simulink model "s0513_eARCmechfailflag_simplecomparison"  (R2021a)
settings: Solver=VariableStepAuto  StartTime=0.0  StopTime=10.0  RelTol=1e-3
libraries: CarMaker4SL x4
settings Model: Creator=jason  LastModifiedBy=jason

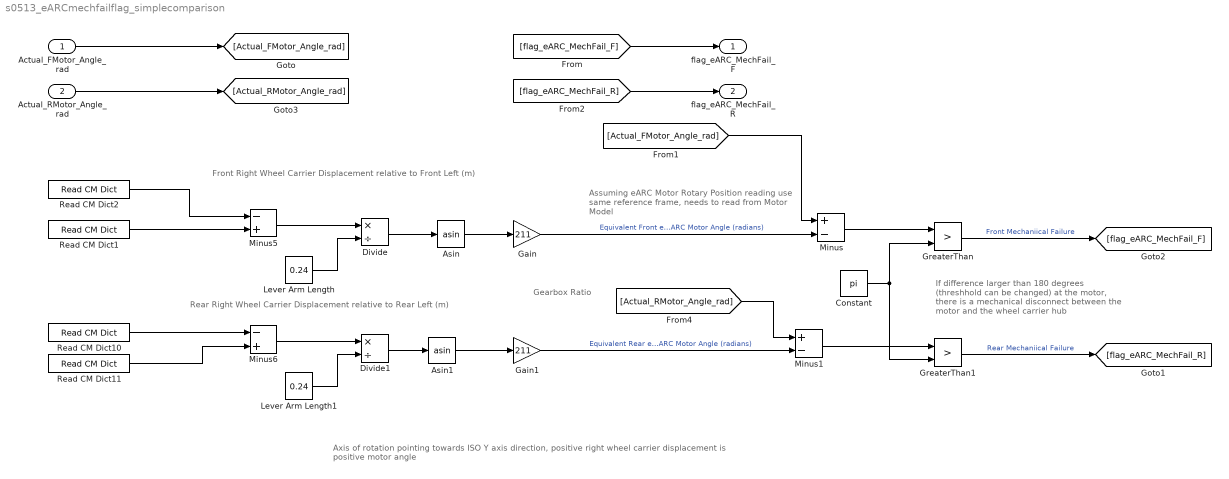
== system s0513_eARCmechfailflag_simplecomparison ==
  note: If difference larger than 180 degrees (threshhold can be changed) at the motor, there is a mechanical disconnect between the motor and the wheel carrier hub
  note: Assuming eARC Motor Rotary Position reading
      | use same reference frame, needs to read from Motor Model
  note: Axis of rotation pointing towards ISO Y axis direction, positive right wheel carrier displacement is positive motor angle
  note: Gearbox Ratio
  note: Rear Right Wheel Carrier Displacement relative to Rear Left (m)
  note: Front Right Wheel Carrier Displacement relative to Front Left (m)
  Actual_FMotor_Angle_rad : Inport
  Actual_RMotor_Angle_rad : Inport  Port=2
  Asin : Trigonometry  Operator=asin
  Asin1 : Trigonometry  Operator=asin
  Constant : Constant  Value=pi
  Divide : Product  Inputs=*/
  Divide1 : Product  Inputs=*/
  Gain : Gain  Gain=211
  Gain1 : Gain  Gain=211
  GreaterThan : RelationalOperator  Operator=>  OutDataTypeStr=boolean  RndMeth=Simplest
  GreaterThan1 : RelationalOperator  Operator=>  OutDataTypeStr=boolean  RndMeth=Simplest
  Lever Arm Length : Constant  Value=0.24
  Lever Arm Length1 : Constant  Value=0.24
  Minus : Sum  Inputs=+-
  Minus1 : Sum  Inputs=+-
  Minus5 : Sum  Inputs=-+
  Minus6 : Sum  Inputs=-+
  Read CM Dict1 : CarMaker4SL/Read CM Dict  xname=Car.CFR.q0  xsync=off  xstime=Continuous
  Read CM Dict10 : CarMaker4SL/Read CM Dict  xname=Car.CRL.q0  xsync=off  xstime=Continuous
  Read CM Dict11 : CarMaker4SL/Read CM Dict  xname=Car.CRR.q0  xsync=off  xstime=Continuous
  Read CM Dict2 : CarMaker4SL/Read CM Dict  xname=Car.CFL.q0  xsync=off  xstime=Continuous
  flag_eARC_MechFail_F : Outport
  flag_eARC_MechFail_R : Outport  Port=2
  wires:
  Minus6/1 -> Divide1/1
  Gain/1 -> Minus/2  "Equivalent Front eARC Motor Angle (radians)"
  Constant/1 -> GreaterThan1/2, GreaterThan/2
  Read CM Dict1/1 -> Minus5/2
  GreaterThan1/1 -> [flag_eARC_MechFail_R]  "Rear Mechaniical Failure"
  Gain1/1 -> Minus1/2  "Equivalent Rear eARC Motor Angle (radians)"
  GreaterThan/1 -> [flag_eARC_MechFail_F]  "Front Mechaniical Failure"
  Minus1/1 -> GreaterThan1/1
  [Actual_FMotor_Angle_rad] -> Minus/1
  [Actual_RMotor_Angle_rad] -> Minus1/1
  Lever Arm Length1/1 -> Divide1/2
  Lever Arm Length/1 -> Divide/2
  Divide1/1 -> Asin1/1
  Minus5/1 -> Divide/1
  Minus/1 -> GreaterThan/1
  Divide/1 -> Asin/1
  Read CM Dict2/1 -> Minus5/1
  Asin1/1 -> Gain1/1
  Asin/1 -> Gain/1
  Read CM Dict10/1 -> Minus6/1
  Read CM Dict11/1 -> Minus6/2
  Actual_FMotor_Angle_rad/1 -> [Actual_FMotor_Angle_rad]
  Actual_RMotor_Angle_rad/1 -> [Actual_RMotor_Angle_rad]
  [flag_eARC_MechFail_F] -> flag_eARC_MechFail_F/1
  [flag_eARC_MechFail_R] -> flag_eARC_MechFail_R/1
